simulink library "lib_OBC"  (R2017a)
settings: Solver=VariableStepAuto  StartTime=0.0  StopTime=10.0  RelTol=1e-3
undefined symbols (not defined in the file): obc
libraries: EC2_libraries x4
settings Model: Creator=Di Russo  LastModifiedBy=Vraj M

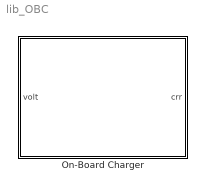
== system lib_OBC ==
  On-Board Charger : Subsystem
      mask Display:
      | image('Images/OBC.jpg')
      | color('red');
      | port_label('Input',1,'Volt')
      | port_label('Output',1,'Crr')

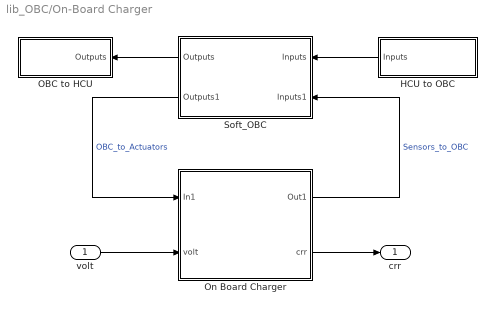
== system lib_OBC/On-Board Charger ==
  volt : Inport
  HCU to OBC : Subsystem
  OBC to HCU : Subsystem
  On Board Charger : Subsystem
      mask Display:
      | image('Images/OBC.jpg')
      | color('red');
      | port_label('Input',1,'Volt')
      | port_label('Output',1,'Crr')
  Soft_OBC : Subsystem
      mask Display: image('SoftECU.jpg')
  crr : Outport
  wires:
  Soft_OBC/2(Outputs1) -> On Board Charger/1("In1 ")  "OBC_to_Actuators"
  On Board Charger/1(Out1) -> Soft_OBC/2(Inputs1)  "Sensors_to_OBC"
  Soft_OBC/1(Outputs) -> OBC to HCU/1(Outputs)
  HCU to OBC/1(Inputs) -> Soft_OBC/1(Inputs)
  On Board Charger/2(crr) -> crr/1
  volt/1 -> On Board Charger/2(volt)

== system lib_OBC/On-Board Charger/HCU to OBC ==
  Bus Creator1 : BusCreator  Inputs=2
  CAN_fromHCU : Subsystem
  Digital_fromHCU : Subsystem
  Inputs : Outport
  wires:
  Bus Creator1/1 -> Inputs/1
  CAN_fromHCU/1(Outputs) -> Bus Creator1/1
  Digital_fromHCU/1(Outputs) -> Bus Creator1/2

== system lib_OBC/On-Board Charger/OBC to HCU ==
  Outputs : Inport
  Bus Selector : BusSelector  OutputSignals=OBC_CAN
  tag scope: OBC_to_HCU=global
  wires:
  Outputs/1 -> Bus Selector/1
  Bus Selector/1 -> [OBC_to_HCU]  "<OBC_CAN>"

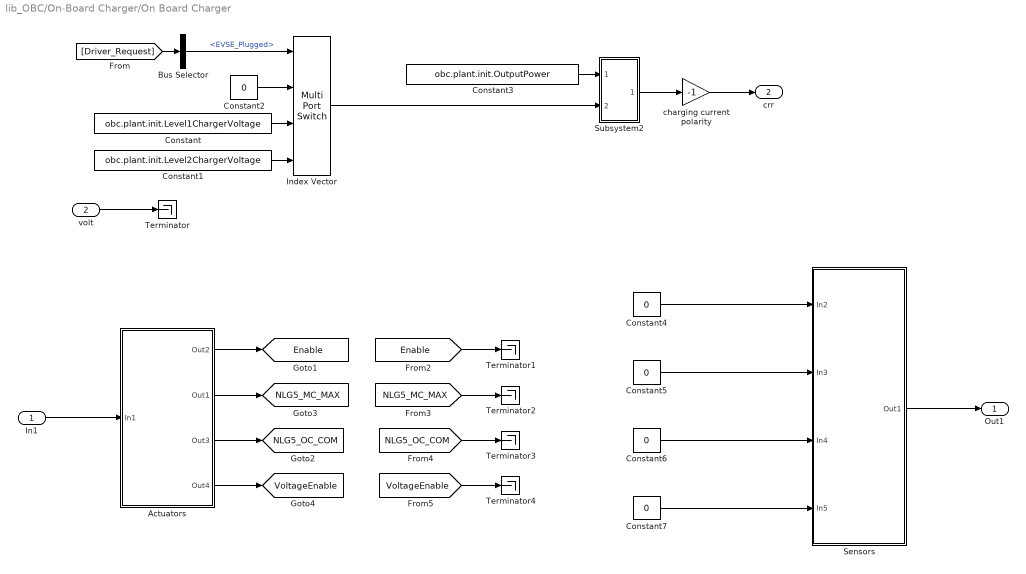
== system lib_OBC/On-Board Charger/On Board Charger ==
  "In1 " : Inport
  volt : Inport  Port=2
  " Actuators" : Subsystem
  Bus Selector : BusSelector  OutputSignals=EVSE_Plugged
  Constant : Constant  Value=obc.plant.init.Level1ChargerVoltage
  Constant1 : Constant  Value=obc.plant.init.Level2ChargerVoltage
  Constant{2,4..7} (5 alike) : Constant  Value=0
  Constant3 : Constant  Value=obc.plant.init.OutputPower
  Index Vector : MultiPortSwitch  DataPortOrder=Zero-based contiguous  zeroidx=on
  Sensors : Subsystem
  Subsystem2 : Subsystem
      mask Display: disp('divider')
  Terminator{,1..4} (5 alike) : Terminator
  "charging current polarity " : Gain  Gain=-1
  Out1 : Outport
  crr : Outport  Port=2
  tag scope: Enable=global, NLG5_MC_MAX=global, NLG5_OC_COM=global, VoltageEnable=global
  wires:
  [VoltageEnable] -> Terminator4/1
  [NLG5_OC_COM] -> Terminator3/1
  [NLG5_MC_MAX] -> Terminator2/1
  [Enable] -> Terminator1/1
  " Actuators"/4(Out4) -> [VoltageEnable]
  " Actuators"/3(Out3) -> [NLG5_OC_COM]
  " Actuators"/2(Out1) -> [NLG5_MC_MAX]
  " Actuators"/1(Out2) -> [Enable]
  "In1 "/1 -> " Actuators"/1(In1)
  Constant5/1 -> Sensors/2(In3)
  Sensors/1(Out1) -> Out1/1
  Constant7/1 -> Sensors/4(In5)
  Constant6/1 -> Sensors/3(In4)
  Constant4/1 -> Sensors/1(In2)
  Index Vector/1 -> Subsystem2/2(In2)
  Bus Selector/1 -> Index Vector/1  "<EVSE_Plugged>"
  [Driver_Request] -> Bus Selector/1
  Constant1/1 -> Index Vector/4
  Constant/1 -> Index Vector/3
  Constant2/1 -> Index Vector/2
  Subsystem2/1(Out1) -> "charging current polarity "/1
  volt/1 -> Terminator/1
  Constant3/1 -> Subsystem2/1(In1)
  "charging current polarity "/1 -> crr/1

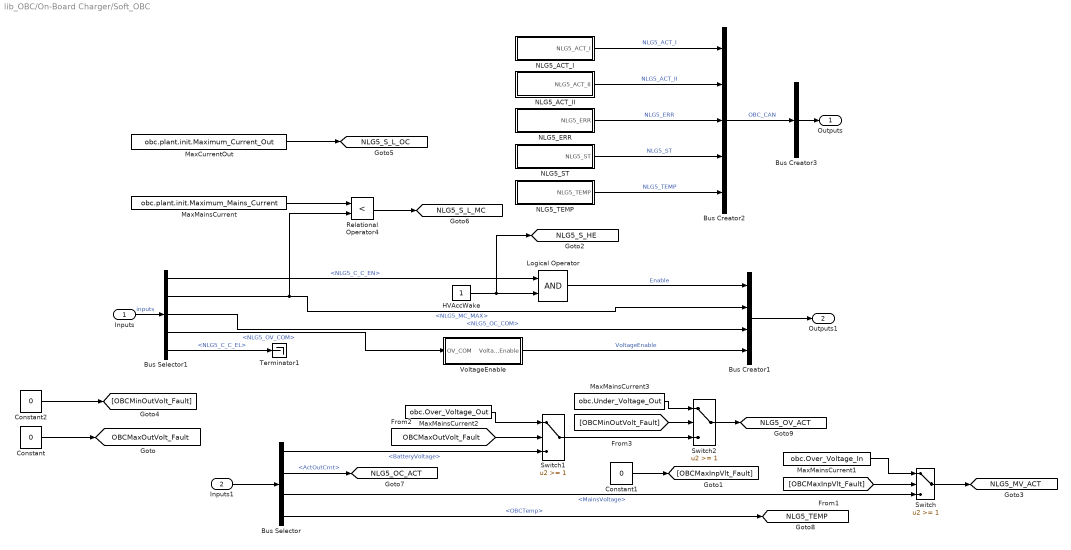
== system lib_OBC/On-Board Charger/Soft_OBC ==
  Inputs : Inport
  Inputs1 : Inport  Port=2
  Bus Creator1 : BusCreator  Inputs=4
  Bus Creator2 : BusCreator  Inputs=5
  Bus Creator3 : BusCreator  Inputs=1
  Bus Selector : BusSelector  OutputSignals=BatteryVoltage,ActOutCrnt,MainsVoltage,OBCTemp
  Bus Selector1 : BusSelector  OutputSignals=to HV_CAN.NLG5_CTL.NLG5_C_C_EN,to HV_CAN.NLG5_CTL.NLG5_MC_MAX,to HV_CAN.NLG5_CTL.NLG5_OC_COM,to HV_CAN.NLG5_CTL.NLG5_OV_COM,to HV_CAN.NLG5_CTL.NLG5_C_C_EL
  Constant : Constant  Value=0
  Constant1 : Constant  Value=0
  Constant2 : Constant  Value=0
  HVAccWake : Constant
  Logical Operator : Logic  AllPortsSameDT=off  OutDataTypeStr=boolean
  MaxCurrentOut : Constant  Value=obc.plant.init.Maximum_Current_Out
  MaxMainsCurrent : Constant  Value=obc.plant.init.Maximum_Mains_Current
  MaxMainsCurrent1 : Constant  Value=obc.Over_Voltage_In
  MaxMainsCurrent2 : Constant  Value=obc.Over_Voltage_Out
  MaxMainsCurrent3 : Constant  Value=obc.Under_Voltage_Out
  NLG5_ACT_I : Subsystem
  NLG5_ACT_II : Subsystem
  NLG5_ERR : Subsystem
  NLG5_ST : Subsystem
  NLG5_TEMP : Subsystem
  Relational Operator4 : RelationalOperator  Operator=<  OutDataTypeStr=boolean  RndMeth=Nearest
  Switch : Switch  Threshold=1
  Switch1 : Switch  Threshold=1
  Switch2 : Switch  Threshold=1
  Terminator1 : Terminator
  VoltageEnable : Subsystem
  Outputs : Outport
  Outputs1 : Outport  Port=2
  tag scope: NLG5_MV_ACT=global, NLG5_OC_ACT=global, NLG5_OV_ACT=global, NLG5_S_HE=global, NLG5_S_L_MC=global, NLG5_S_L_OC=global, NLG5_TEMP=global, OBCMaxOutVolt_Fault=global
  wires:
  Constant2/1 -> [OBCMinOutVolt_Fault]
  Constant1/1 -> [OBCMaxInpVlt_Fault]
  Constant/1 -> [OBCMaxOutVolt_Fault]
  Bus Selector1/4 -> VoltageEnable/1(OV_COM)  "<NLG5_OV_COM>"
  Bus Selector1/3 -> Bus Creator1/3  "<NLG5_OC_COM>"
  Bus Selector1/2 -> Bus Creator1/2, Relational Operator4/2  "<NLG5_MC_MAX>"
  HVAccWake/1 -> Logical Operator/2, [NLG5_S_HE]
  MaxMainsCurrent3/1 -> Switch2/1
  [OBCMinOutVolt_Fault] -> Switch2/2
  Switch2/1 -> [NLG5_OV_ACT]
  Switch1/1 -> Switch2/3
  Bus Selector/4 -> [NLG5_TEMP]  "<OBCTemp>"
  Bus Selector/1 -> Switch1/3  "<BatteryVoltage>"
  MaxMainsCurrent2/1 -> Switch1/1
  [OBCMaxOutVolt_Fault] -> Switch1/2
  Switch/1 -> [NLG5_MV_ACT]
  MaxMainsCurrent1/1 -> Switch/1
  Bus Selector/3 -> Switch/3  "<MainsVoltage>"
  [OBCMaxInpVlt_Fault] -> Switch/2
  Bus Selector/2 -> [NLG5_OC_ACT]  "<ActOutCrnt>"
  Relational Operator4/1 -> [NLG5_S_L_MC]
  MaxMainsCurrent/1 -> Relational Operator4/1
  MaxCurrentOut/1 -> [NLG5_S_L_OC]
  Logical Operator/1 -> Bus Creator1/1  "Enable"
  Bus Creator1/1 -> Outputs1/1
  Inputs1/1 -> Bus Selector/1
  NLG5_ACT_I/1(NLG5_ACT_I) -> Bus Creator2/1  "NLG5_ACT_I"
  Bus Creator2/1 -> Bus Creator3/1  "OBC_CAN"
  Bus Creator3/1 -> Outputs/1
  NLG5_ACT_II/1(NLG5_ACT_II) -> Bus Creator2/2  "NLG5_ACT_II"
  NLG5_ERR/1(NLG5_ERR) -> Bus Creator2/3  "NLG5_ERR"
  NLG5_TEMP/1(NLG5_TEMP) -> Bus Creator2/5  "NLG5_TEMP"
  Inputs/1 -> Bus Selector1/1  "inputs"
  Bus Selector1/1 -> Logical Operator/1  "<NLG5_C_C_EN>"
  Bus Selector1/5 -> Terminator1/1  "<NLG5_C_C_EL>"
  VoltageEnable/1(VoltageEnable) -> Bus Creator1/4  "VoltageEnable"
  NLG5_ST/1(NLG5_ST) -> Bus Creator2/4  "NLG5_ST"

== system lib_OBC/On-Board Charger/HCU to OBC/CAN_fromHCU ==
  Outputs : Outport
  wires:
  [HCU_to_HV_CAN] -> Outputs/1

== system lib_OBC/On-Board Charger/HCU to OBC/Digital_fromHCU ==
  Outputs : Outport
  wires:
  [Digital] -> Outputs/1

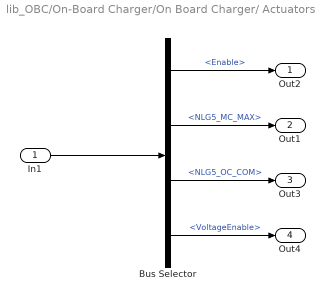
== system lib_OBC/On-Board Charger/On Board Charger/ Actuators ==
  In1 : Inport
  Bus Selector : BusSelector  OutputSignals=Enable,NLG5_MC_MAX,NLG5_OC_COM,VoltageEnable
  Out2 : Outport
  Out1 : Outport  Port=2
  Out3 : Outport  Port=3
  Out4 : Outport  Port=4
  wires:
  Bus Selector/4 -> Out4/1  "<VoltageEnable>"
  Bus Selector/3 -> Out3/1  "<NLG5_OC_COM>"
  Bus Selector/2 -> Out1/1  "<NLG5_MC_MAX>"
  In1/1 -> Bus Selector/1
  Bus Selector/1 -> Out2/1  "<Enable>"

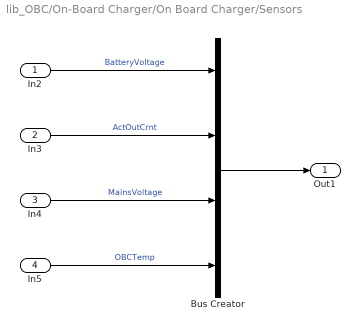
== system lib_OBC/On-Board Charger/On Board Charger/Sensors ==
  In2 : Inport
  In3 : Inport  Port=2
  In4 : Inport  Port=3
  In5 : Inport  Port=4
  Bus Creator : BusCreator  Inputs=4
  Out1 : Outport
  wires:
  Bus Creator/1 -> Out1/1
  In2/1 -> Bus Creator/1  "BatteryVoltage"
  In4/1 -> Bus Creator/3  "MainsVoltage"
  In5/1 -> Bus Creator/4  "OBCTemp"
  In3/1 -> Bus Creator/2  "ActOutCrnt"

== system lib_OBC/On-Board Charger/On Board Charger/Subsystem2 ==
  In1 : Inport
  In2 : Inport  Port=2
  Fcn : Fcn  Expr=u[1]/(u[2]+eps)*(u[2]!=0)
  Mux : Mux  Inputs=2
  Out1 : Outport
  wires:
  Mux/1 -> Fcn/1
  In1/1 -> Mux/1
  Fcn/1 -> Out1/1
  In2/1 -> Mux/2

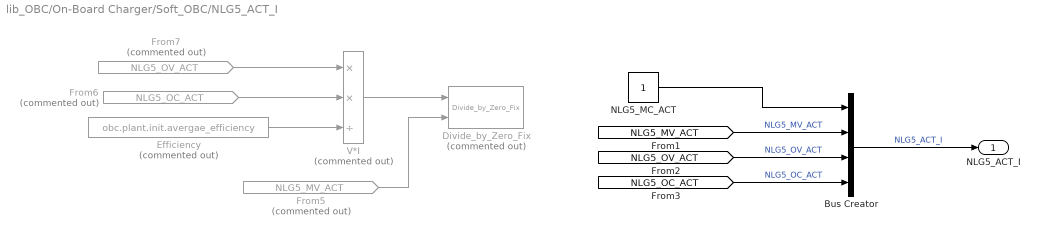
== system lib_OBC/On-Board Charger/Soft_OBC/NLG5_ACT_I ==
  Bus Creator : BusCreator  Inputs=4
  Divide_by_Zero_Fix : EC2_libraries/Divide_by_Zero_Fix  Commented=on
  Efficiency : Constant  Commented=on  Value=obc.plant.init.avergae_efficiency
  From5 : From  Commented=on  GotoTag=NLG5_MV_ACT  TagVisibility=global
  From6 : From  Commented=on  GotoTag=NLG5_OC_ACT  TagVisibility=global
  From7 : From  Commented=on  GotoTag=NLG5_OV_ACT  TagVisibility=global
  NLG5_MC_ACT : Constant
  V*I : Product  Commented=on  Inputs=**/  RndMeth=Zero
  NLG5_ACT_I : Outport
  wires:
  NLG5_MC_ACT/1 -> Bus Creator/1
  From7/1 -> V*I/1
  From6/1 -> V*I/2
  Bus Creator/1 -> NLG5_ACT_I/1  "NLG5_ACT_I"
  [NLG5_MV_ACT] -> Bus Creator/2  "NLG5_MV_ACT"
  [NLG5_OC_ACT] -> Bus Creator/4  "NLG5_OC_ACT"
  [NLG5_OV_ACT] -> Bus Creator/3  "NLG5_OV_ACT"
  Efficiency/1 -> V*I/3
  V*I/1 -> Divide_by_Zero_Fix/1
  From5/1 -> Divide_by_Zero_Fix/2

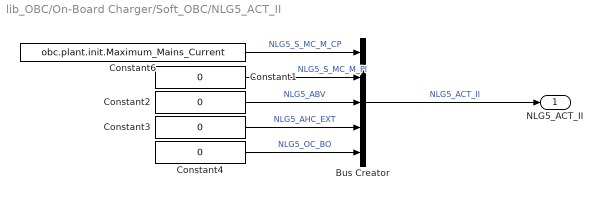
== system lib_OBC/On-Board Charger/Soft_OBC/NLG5_ACT_II ==
  Bus Creator : BusCreator  Inputs=5
  Constant{1..4} (4 alike) : Constant  Value=0
  Constant6 : Constant  Value=obc.plant.init.Maximum_Mains_Current
  NLG5_ACT_II : Outport
  wires:
  Constant2/1 -> Bus Creator/3  "NLG5_ABV"
  Constant3/1 -> Bus Creator/4  "NLG5_AHC_EXT"
  Constant1/1 -> Bus Creator/2  "NLG5_S_MC_M_PI"
  Constant6/1 -> Bus Creator/1  "NLG5_S_MC_M_CP"
  Bus Creator/1 -> NLG5_ACT_II/1  "NLG5_ACT_II"
  Constant4/1 -> Bus Creator/5  "NLG5_OC_BO"

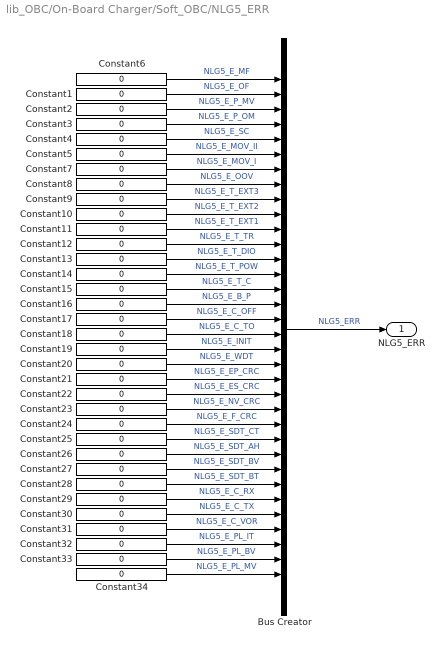
== system lib_OBC/On-Board Charger/Soft_OBC/NLG5_ERR ==
  Bus Creator : BusCreator  Inputs=34
  Constant{1..34} (34 alike) : Constant  Value=0
  NLG5_ERR : Outport
  wires:
  Constant4/1 -> Bus Creator/5  "NLG5_E_SC"
  Bus Creator/1 -> NLG5_ERR/1  "NLG5_ERR"
  Constant6/1 -> Bus Creator/1  "NLG5_E_MF"
  Constant1/1 -> Bus Creator/2  "NLG5_E_OF"
  Constant3/1 -> Bus Creator/4  "NLG5_E_P_OM"
  Constant2/1 -> Bus Creator/3  "NLG5_E_P_MV"
  Constant5/1 -> Bus Creator/6  "NLG5_E_MOV_II"
  Constant7/1 -> Bus Creator/7  "NLG5_E_MOV_I"
  Constant8/1 -> Bus Creator/8  "NLG5_E_OOV"
  Constant9/1 -> Bus Creator/9  "NLG5_E_T_EXT3"
  Constant10/1 -> Bus Creator/10  "NLG5_E_T_EXT2"
  Constant11/1 -> Bus Creator/11  "NLG5_E_T_EXT1"
  Constant12/1 -> Bus Creator/12  "NLG5_E_T_TR"
  Constant13/1 -> Bus Creator/13  "NLG5_E_T_DIO"
  Constant14/1 -> Bus Creator/14  "NLG5_E_T_POW"
  Constant15/1 -> Bus Creator/15  "NLG5_E_T_C"
  Constant16/1 -> Bus Creator/16  "NLG5_E_B_P"
  Constant17/1 -> Bus Creator/17  "NLG5_E_C_OFF"
  Constant18/1 -> Bus Creator/18  "NLG5_E_C_TO"
  Constant19/1 -> Bus Creator/19  "NLG5_E_INIT"
  Constant20/1 -> Bus Creator/20  "NLG5_E_WDT"
  Constant21/1 -> Bus Creator/21  "NLG5_E_EP_CRC"
  Constant22/1 -> Bus Creator/22  "NLG5_E_ES_CRC"
  Constant23/1 -> Bus Creator/23  "NLG5_E_NV_CRC"
  Constant24/1 -> Bus Creator/24  "NLG5_E_F_CRC"
  Constant25/1 -> Bus Creator/25  "NLG5_E_SDT_CT"
  Constant26/1 -> Bus Creator/26  "NLG5_E_SDT_AH"
  Constant27/1 -> Bus Creator/27  "NLG5_E_SDT_BV"
  Constant28/1 -> Bus Creator/28  "NLG5_E_SDT_BT"
  Constant29/1 -> Bus Creator/29  "NLG5_E_C_RX"
  Constant30/1 -> Bus Creator/30  "NLG5_E_C_TX"
  Constant31/1 -> Bus Creator/31  "NLG5_E_C_VOR"
  Constant32/1 -> Bus Creator/32  "NLG5_E_PL_IT"
  Constant33/1 -> Bus Creator/33  "NLG5_E_PL_BV"
  Constant34/1 -> Bus Creator/34  "NLG5_E_PL_MV"

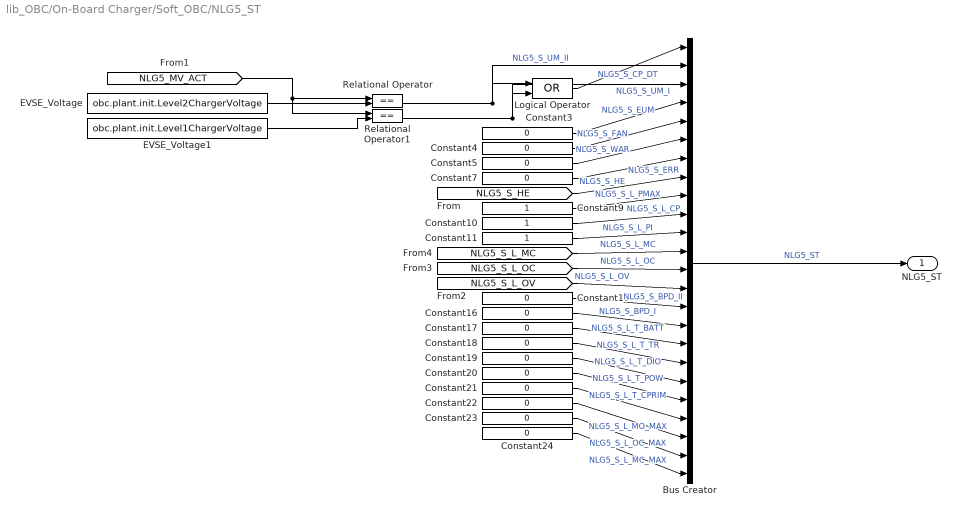
== system lib_OBC/On-Board Charger/Soft_OBC/NLG5_ST ==
  Bus Creator : BusCreator  Inputs=24
  Constant10 : Constant
  Constant11 : Constant
  Constant{3..5,7,15..24} (14 alike) : Constant  Value=0
  Constant9 : Constant
  EVSE_Voltage : Constant  Value=obc.plant.init.Level2ChargerVoltage
  EVSE_Voltage1 : Constant  Value=obc.plant.init.Level1ChargerVoltage
  Logical Operator : Logic  Operator=OR  AllPortsSameDT=off  OutDataTypeStr=boolean
  Relational Operator : RelationalOperator  Operator===  OutDataTypeStr=boolean  RndMeth=Nearest
  Relational Operator1 : RelationalOperator  Operator===  OutDataTypeStr=boolean  RndMeth=Nearest
  NLG5_ST : Outport
  wires:
  Constant24/1 -> Bus Creator/24  "NLG5_S_L_MC_MAX"
  Constant23/1 -> Bus Creator/23  "NLG5_S_L_OC_MAX"
  Constant22/1 -> Bus Creator/22  "NLG5_S_L_MO_MAX"
  Constant21/1 -> Bus Creator/21  "NLG5_S_L_T_CPRIM"
  Constant20/1 -> Bus Creator/20  "NLG5_S_L_T_POW"
  Constant19/1 -> Bus Creator/19  "NLG5_S_L_T_DIO"
  Constant18/1 -> Bus Creator/18  "NLG5_S_L_T_TR"
  Constant17/1 -> Bus Creator/17  "NLG5_S_L_T_BATT"
  Constant16/1 -> Bus Creator/16  "NLG5_S_BPD_I"
  Constant15/1 -> Bus Creator/15  "NLG5_S_BPD_II"
  [NLG5_S_L_OV] -> Bus Creator/14  "NLG5_S_L_OV"
  [NLG5_S_L_OC] -> Bus Creator/13  "NLG5_S_L_OC"
  [NLG5_S_L_MC] -> Bus Creator/12  "NLG5_S_L_MC"
  Constant11/1 -> Bus Creator/11  "NLG5_S_L_PI"
  Constant10/1 -> Bus Creator/10  "NLG5_S_L_CP"
  Constant9/1 -> Bus Creator/9  "NLG5_S_L_PMAX"
  [NLG5_S_HE] -> Bus Creator/8  "NLG5_S_HE"
  Constant7/1 -> Bus Creator/7  "NLG5_S_ERR"
  Constant5/1 -> Bus Creator/6  "NLG5_S_WAR"
  Relational Operator1/1 -> Logical Operator/2, Bus Creator/3  "NLG5_S_UM_I"
  Constant3/1 -> Bus Creator/4  "NLG5_S_EUM"
  Relational Operator/1 -> Logical Operator/1, Bus Creator/2  "NLG5_S_UM_II"
  Logical Operator/1 -> Bus Creator/1  "NLG5_S_CP_DT"
  Bus Creator/1 -> NLG5_ST/1  "NLG5_ST"
  Constant4/1 -> Bus Creator/5  "NLG5_S_FAN"
  [NLG5_MV_ACT] -> Relational Operator/1, Relational Operator1/1
  EVSE_Voltage/1 -> Relational Operator/2
  EVSE_Voltage1/1 -> Relational Operator1/2

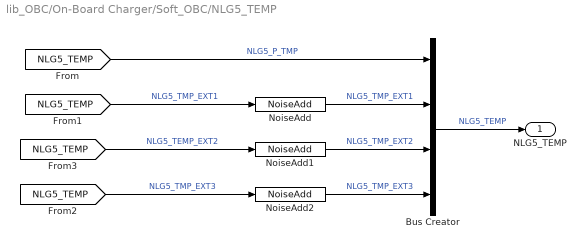
== system lib_OBC/On-Board Charger/Soft_OBC/NLG5_TEMP ==
  Bus Creator : BusCreator  Inputs=4
  NoiseAdd : EC2_libraries/NoiseAdd  variance=0  seed=0
  NoiseAdd1 : EC2_libraries/NoiseAdd  variance=0  seed=0
  NoiseAdd2 : EC2_libraries/NoiseAdd  variance=0  seed=0
  NLG5_TEMP : Outport
  wires:
  NoiseAdd2/1 -> Bus Creator/4  "NLG5_TMP_EXT3"
  NoiseAdd1/1 -> Bus Creator/3  "NLG5_TMP_EXT2"
  NoiseAdd/1 -> Bus Creator/2  "NLG5_TMP_EXT1"
  [NLG5_TEMP] -> NoiseAdd1/1  "NLG5_TEMP_EXT2"
  [NLG5_TEMP] -> NoiseAdd2/1  "NLG5_TMP_EXT3"
  [NLG5_TEMP] -> NoiseAdd/1  "NLG5_TMP_EXT1"
  [NLG5_TEMP] -> Bus Creator/1  "NLG5_P_TMP"
  Bus Creator/1 -> NLG5_TEMP/1  "NLG5_TEMP"

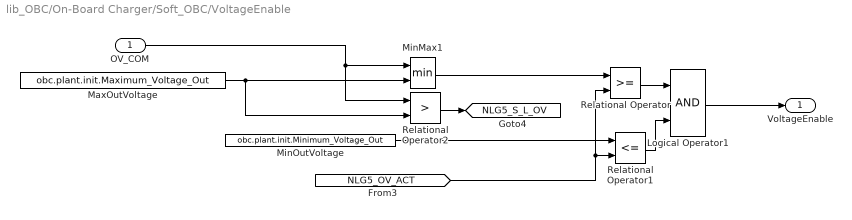
== system lib_OBC/On-Board Charger/Soft_OBC/VoltageEnable ==
  OV_COM : Inport
  Logical Operator1 : Logic  AllPortsSameDT=off  OutDataTypeStr=boolean
  MaxOutVoltage : Constant  Value=obc.plant.init.Maximum_Voltage_Out
  MinMax1 : MinMax  Inputs=2
  MinOutVoltage : Constant  Value=obc.plant.init.Minimum_Voltage_Out
  Relational Operator : RelationalOperator  OutDataTypeStr=boolean  RndMeth=Nearest
  Relational Operator1 : RelationalOperator  Operator=<=  OutDataTypeStr=boolean  RndMeth=Nearest
  Relational Operator2 : RelationalOperator  Operator=>  OutDataTypeStr=boolean  RndMeth=Nearest
  VoltageEnable : Outport
  tag scope: NLG5_S_L_OV=global
  wires:
  [NLG5_OV_ACT] -> Relational Operator1/2, Relational Operator/2
  Logical Operator1/1 -> VoltageEnable/1
  Relational Operator2/1 -> [NLG5_S_L_OV]
  MinOutVoltage/1 -> Relational Operator1/1
  Relational Operator/1 -> Logical Operator1/1
  Relational Operator1/1 -> Logical Operator1/2
  OV_COM/1 -> Relational Operator2/1, MinMax1/1
  MaxOutVoltage/1 -> Relational Operator2/2, MinMax1/2
  MinMax1/1 -> Relational Operator/1
